simulink model "sound_fal"  (Simulink 10.1)
settings: Solver=FixedStepAuto  StartTime=0.0  StopTime=60  FixedStep=fixedStep  MaxStep=0.2  RelTol=1e-3
values from neighbouring files (symbols this model uses):
  configSoundSource = [1 58]    [garbageDisposalInit.m]
  disSoundSource = disGarbageDisposal    [garbageDisposalInit.m]
settings Model: Creator=lixuansong  LastModifiedBy=ozgurozmen
settings DataIOCC: SaveOutput=off  SignalLogging=off  DSMLogging=off  SaveTime=off
settings OptimizationCC: LifeSpan=auto
settings DebuggingCC: UnderspecifiedInitializationDetection=Simplified  MergeDetectMultiDrivingBlocksExec=error  SFUnexpectedBacktrackingDiag=error  SFNoUnconditionalDefaultTransitionDiag=error  SFExecutionAtInitializationDiag=warning  ArithmeticOperatorsInVariantConditions=error
settings HardwareCC: ProdBitPerPointer=64  ProdBitPerSizeT=64  ProdBitPerPtrDiffT=64  ProdLargestAtomicFloat=Float  ProdIntDivRoundTo=Zero  ProdEndianess=LittleEndian  ProdWordSize=64  ProdHWDeviceType=Intel->x86-64 (Windows64)
settings ModelReferenceCC: PropagateSignalLabelsOutOfModel=on
settings SFSimCC: SimUseLocalCustomCode=on  CustomCodeUndefinedFunction=FilterOut
settings RTWCC: RTWUseLocalCustomCode=on
settings CodeAppCC: StateflowObjectComments=off
settings GRTTargetCC: TargetLangStandard=C99 (ISO)  CombineOutputUpdateFcns=on  GRTInterface=off
settings ConfigComp: CovMetricSettings=dwe  CovHtmlReporting=off  CovSaveCumulativeToWorkspaceVar=off  CovSaveSingleToWorkspaceVar=off  CovExternalEMLEnable=on

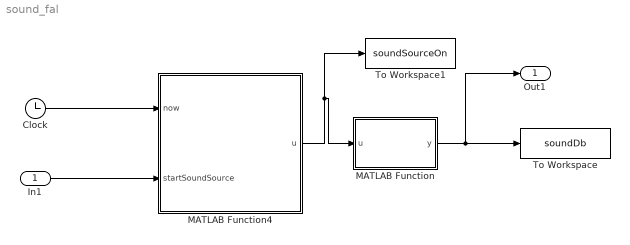
== system sound_fal ==
  In1 : Inport
  Clock : Clock
  MATLAB Function : MATLAB Function  TreatAsAtomicUnit=on
  MATLAB Function4 : MATLAB Function  TreatAsAtomicUnit=on
  To Workspace : ToWorkspace  VariableName=soundDb  SampleTime=-1
  To Workspace1 : ToWorkspace  VariableName=soundSourceOn  SampleTime=-1
  Out1 : Outport
  wires:
  MATLAB Function4/1(u) -> To Workspace1/1, MATLAB Function/1(u)
  Clock/1 -> MATLAB Function4/1(now)
  In1/1 -> MATLAB Function4/2(startSoundSource)
  MATLAB Function/1(y) -> Out1/1, To Workspace/1

== matlab function MATLAB Function ==
  data: u input double; y output double; disSoundSource parameter double; configSoundSource parameter double
function y = calSound(u, disSoundSource,configSoundSource)

dis0=configSoundSource(1);%distance in configuration
db0=configSoundSource(2);%db in configuration

if u==1
    y=db0-log2(disSoundSource/dis0)*6;
else
    y=0;
end

== matlab function MATLAB Function4 ==
  data: u output double; now input double; timeSoundSource parameter double; startSoundSource input double
function u = controlSoundSource(now,timeSoundSource, startSoundSource)
if now>=startSoundSource && now<=startSoundSource+timeSoundSource
    u=1;
else
    u=0;
end
